simulink model "LQGR_Complete"  (R2021a)
settings: Solver=VariableStepAuto  StartTime=0.0  StopTime=10.0  RelTol=1e-3
values from neighbouring files (symbols this model uses):
  A_ct = sysest_ct.A    [LQGR_Controller_script.m]
  B_ct = sysest_ct.B    [LQGR_Controller_script.m]
  C_ct = sysest_ct.C    [LQGR_Controller_script.m]
  K_lq = lqr(A_ct, B_ct, Q_lq, R_lq)    [LQGR_Controller_script.m]
  L_kf = lqr(A_ct.', C_ct.', Q_kf, R_kf).'    [LQGR_Controller_script.m]
  v_a_max = 15    [LQGR_Controller_script.m]
  Vd = [0.0001, 0, 0.0001, 0]    [LQGR_Controller_script.m]
undefined symbols (not defined in the file or in its folder): sigbuilder_block
libraries: simulink_extras x2
settings Model: Creator=jesuc  LastModifiedBy=arco

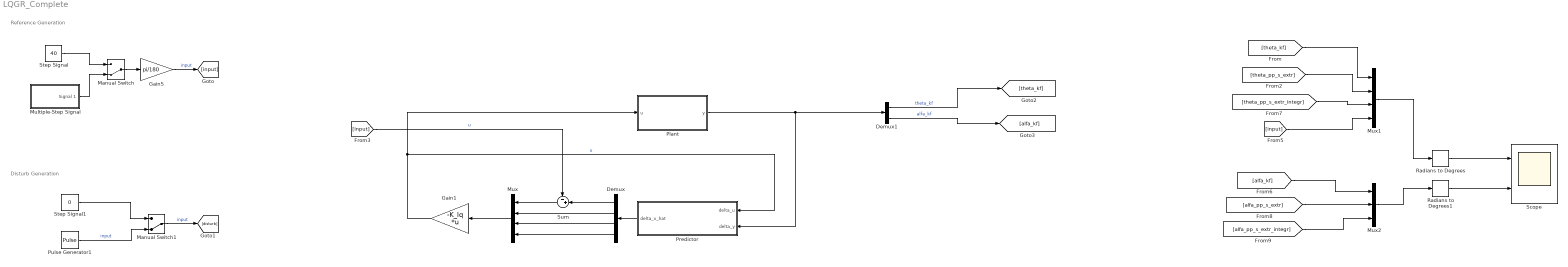
== system LQGR_Complete ==
  note: Reference Generation
  note: Disturb Generation
  Demux : Demux
  Demux1 : Demux  Outputs=2
  Gain1 : Gain  Gain=-K_lq  Multiplication=Matrix(K*u)
  Gain5 : Gain  Gain=pi/180
  Manual Switch : ManualSwitch  CurrentSetting=0
  Manual Switch1 : ManualSwitch  CurrentSetting=0
  Multiple-Step Signal : Subsystem  Tag=STV Subsys  LoadFcn=sigbuilder_block('load');  StartFcn=sigbuilder_block('start');  StopFcn=sigbuilder_block('stop');  ClipboardFcn=sigbuilder_block('clipboard');  mask(Sigbuilder block){tuvar=[0:10]}
      mask help: Simulink:masks:SigbuilderBlock_MD
      mask init:
      | if ~strcmp(get_param(bdroot(gcbh),'SimulationStatus'),'stopped') tuvar = sigbuilder_block('maskInit'); end
      settings: CopyFcn=sigbuilder_block('copy');  DeleteFcn=sigbuilder_block('delete');  ModelCloseFcn=sigbuilder_block('modelClose');  PreSaveFcn=sigbuilder_block('preSave');  PauseFcn=sigbuilder_block('pause');  ContinueFcn=sigbuilder_block('continue');  NameChangeFcn=sigbuilder_block('namechange');  OpenFcn=sigbuilder_block('open',[437.6 199.2 550.4 400 ]);  CloseFcn=sigbuilder_block('close');
      mask Display: plot(0, 0, 100, 100,[2, 2, 32, 32, 2], [68, 8, 8, 68, 68],[32, 2], [38, 38], [32, 19, 2],[53, 60, 44], [32, 17, 17, 2],[16, 16, 31, 31]);txt = getActiveGroup(gcbh);text(2, 100, txt,'verticalAlignment', 'top');
  Mux : Mux
  Mux1 : Mux
  Mux2 : Mux  Inputs=3
  Plant : Subsystem
  Predictor : Subsystem
      settings: PortSchema="{\"entries\":[{\"content\":{\"sides\":[{\"content\":{\"connectorIds\":[\"Out1\"]},\"type\":\"ConnectorPlacement.EquallySpacedRectSide\",\"uuid\":\"cdc36ef1-b9aa-4793-8815-08646de90a91\"},{\"content\":{\"connectorIds\":[\"In1\",\"In2\"],\"side\":\"RIGHT\"},\"type\":\"ConnectorPlacement.EquallySpacedRectSide\",\"uuid\":\"c826576a-106c-43df-aaf0-aa674a969d04\"},{\"content\":{\"connectorIds\":[],\"side\":\"TOP\"},\"type\":\"ConnectorPlacement.EquallySpacedRectSide\",\"uuid\":\"d2200aa9-f6c9-47e5-a9d0-498ec6850ca3\"}]},\"type\":\"ConnectorPlacement.EquallySpacedConnector\",\"uuid\":\"4474187f-41f3-4590-923f-8ea1970bc9fc\"}],\"packageUris\":[\"http://schema.mathworks.com/mf0/Connector/R2020b\"],\"version\":\"1.0\"}"
  Pulse Generator1 : DiscretePulseGenerator  PulseType=Time based  Amplitude=.2  Period=1.5  PulseWidth=5
  Radians to Degrees : simulink_extras/Transformations/Radians to Degrees
  Radians to Degrees1 : simulink_extras/Transformations/Radians to Degrees
  Scope : Scope  NumInputPorts=2
  Step Signal : Constant  Value=40
  Step Signal1 : Constant  Value=0
  Sum : Sum  Inputs=-+|
  wires:
  Demux1/1 -> [theta_kf]  "theta_kf"
  Demux1/2 -> [alfa_kf]  "alfa_kf"
  Mux1/1 -> Radians to Degrees/1
  Multiple-Step Signal/1(Signal 1) -> Manual Switch/2
  Step Signal/1 -> Manual Switch/1
  Manual Switch/1 -> Gain5/1
  Mux2/1 -> Radians to Degrees1/1
  Gain1/1 -> Plant/1(u), Predictor/1(delta_u)  "u"
  Step Signal1/1 -> Manual Switch1/1
  Radians to Degrees/1 -> Scope/1
  Radians to Degrees1/1 -> Scope/2
  Gain5/1 -> [input]  "input"
  Manual Switch1/1 -> [disturb]  "input"
  [input] -> Mux1/4
  [theta_kf] -> Mux1/1
  [theta_pp_s_extr] -> Mux1/2
  [theta_pp_s_extr_integr] -> Mux1/3
  [alfa_kf] -> Mux2/1
  [alfa_pp_s_extr] -> Mux2/2
  [alfa_pp_s_extr_integr] -> Mux2/3
  Pulse Generator1/1 -> Manual Switch1/2  "input"
  Plant/1(y) -> Predictor/2(delta_y), Demux1/1
  Mux/1 -> Gain1/1
  Predictor/1(delta_x_hat) -> Demux/1
  Demux/3 -> Mux/3
  Sum/1 -> Mux/1
  Demux/2 -> Mux/2
  Demux/1 -> Sum/2
  [input] -> Sum/1  "u"
  Demux/4 -> Mux/4

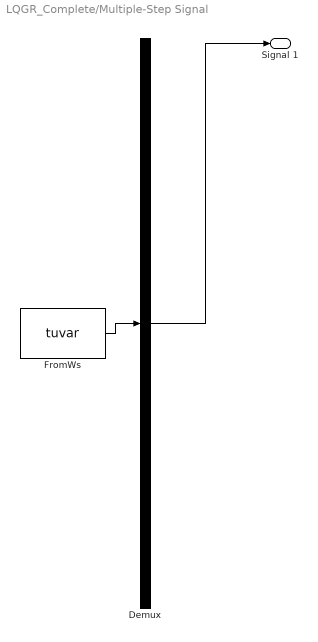
== system LQGR_Complete/Multiple-Step Signal ==
  Demux : Demux  Tag=STV Demux  Outputs=1
      settings: DisplayOption=none
  FromWs : FromWorkspace  Tag=STV FromWs  VariableName=tuvar
      SigBuilderData=|
      | common.afterFinalStr = 'Extrapolate'
      | common.sampleTime = 0
      | dataSet.timeRange = [0 10]
      | dataSet.name = 'Group 1'
      | sbobj.Groups.Name = 'Group 1'
      | sbobj.Groups.Signals.Name = 'Signal 1'
      | sbobj.Groups.Signals.XData = [0 1 1 3 3 5 5 7 7 8.5 8.5 10]
      | sbobj.Groups.Signals.YData = [0.005 0.005 40 40 15 15 -30 -30 0 0 23 23]
  Signal 1 : Outport  Tag=STV Outport
  wires:
  Demux/1 -> Signal 1/1
  FromWs/1 -> Demux/1

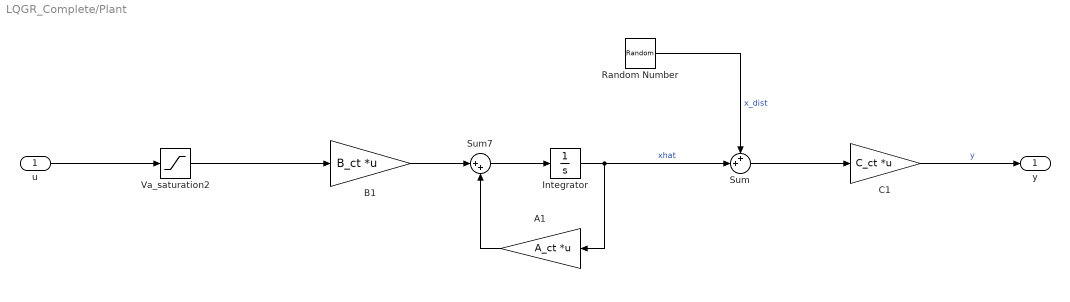
== system LQGR_Complete/Plant ==
  u : Inport
  A1 : Gain  Gain=A_ct  Multiplication=Matrix(K*u) (u vector)
  B1 : Gain  Gain=B_ct  Multiplication=Matrix(K*u) (u vector)
  C1 : Gain  Gain=C_ct  Multiplication=Matrix(K*u) (u vector)
  Integrator : Integrator
  Random Number : RandomNumber  Variance=Vd  SampleTime=0.1
  Sum : Sum  Inputs=++|
  Sum7 : Sum  Inputs=|++
  Va_saturation2 : Saturate  UpperLimit=v_a_max  LowerLimit=-v_a_max
  y : Outport
  wires:
  Sum7/1 -> Integrator/1
  B1/1 -> Sum7/1
  Integrator/1 -> Sum/2, A1/1  "xhat"
  C1/1 -> y/1  "y"
  u/1 -> Va_saturation2/1
  A1/1 -> Sum7/2
  Va_saturation2/1 -> B1/1
  Sum/1 -> C1/1
  Random Number/1 -> Sum/1  "x_dist"

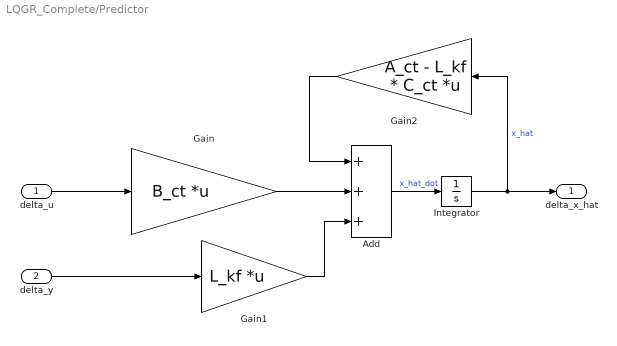
== system LQGR_Complete/Predictor ==
  delta_u : Inport  PortDimensions=1
  delta_y : Inport  Port=2  PortDimensions=2
  Add : Sum  Inputs=+++
  Gain : Gain  Gain=B_ct  Multiplication=Matrix(K*u) (u vector)
  Gain1 : Gain  Gain=L_kf  Multiplication=Matrix(K*u) (u vector)
  Gain2 : Gain  Gain=A_ct - L_kf * C_ct  Multiplication=Matrix(K*u) (u vector)
  Integrator : Integrator
  delta_x_hat : Outport  PortDimensions=4
  wires:
  Gain2/1 -> Add/1
  Integrator/1 -> Gain2/1, delta_x_hat/1  "x_hat"
  Add/1 -> Integrator/1  "x_hat_dot"
  Gain/1 -> Add/2
  delta_u/1 -> Gain/1
  Gain1/1 -> Add/3
  delta_y/1 -> Gain1/1
